simulink model "ConvertFrom_BFloat16_Ex2"  (R2023a)
settings: Solver=VariableStepAuto  StartTime=0.0  StopTime=1  RelTol=1e-3
undefined symbols (not defined in the file): AIE, i, L, ML, nsvh1369, xcvc2602
libraries: aieUtilities x2, vmcUtilities x1, dspsrcs4 x1
settings Model: Creator=sdegala  LastModifiedBy=robg

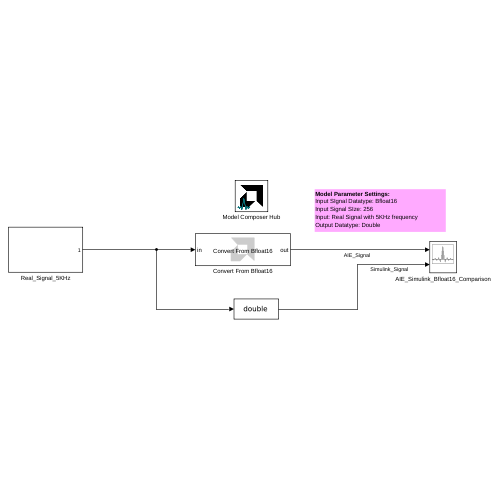
[thumbnail: Simulink's stored preview of the top-level diagram]
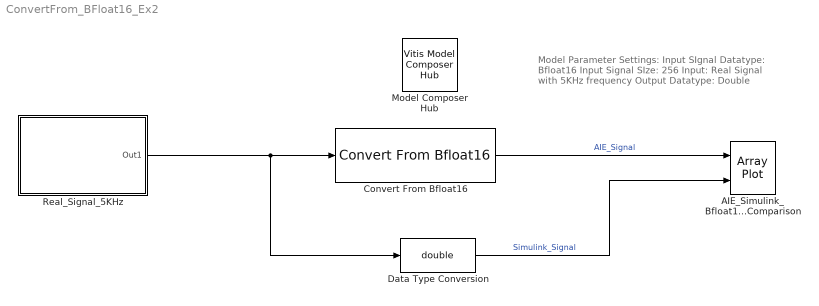
== system ConvertFrom_BFloat16_Ex2 ==
  note: Model Parameter Settings:
      | Input SIgnal Datatype: Bfloat16
      | Input Signal SIze: 256
      | Input: Real Signal with 5KHz frequency
      | Output Datatype: Double
  AIE_Simulink_Bfloat16_Comparison : ArrayPlot  NumInputPorts=2  WindowPosition=[1.000000,6.000000,1274.000000,655.000000,]  ScopeFrameLocation=window  PlotType=Line  YLimits=[-1.25,1.25]  ShowLegend=on  DefaultConfigurationName=dsp.scopes.ArrayPlotBlockSpecification
  Convert From Bfloat16 : aieUtilities/Convert From Bfloat16  OutputDataType=double
  Data Type Conversion : DataTypeConversion  OutDataTypeStr=double  SaturateOnIntegerOverflow=off  RndMeth=Floor
  Model Composer Hub : vmcUtilities/Vitis Model Composer Hub  Tag=genX  CodeGeneration=off  CompilationType=HDLCompilation  ExportTypeV2=IP Catalog  StartColumn=1  NumberOfColumns=1  TargetDirectory=./netlist  exportDesign=off  analyzeDesign=off  validateDesignOnHw=off  ExportType=AI Engines  IpVendor=xilinx.com  IpLibrary=hls  IpVersion=1.0  IpHWLanguage=Verilog  AieCompilerOptions={}  AieSimulatorOptions={}  CreateTestbench=on  TestbenchStackSize=10  RunRtlSim=off  RunCSim=off  RunAieSim=on  AieSimTimeout=50000  RunAieSimProfiling=off  LaunchVitisAnalyzer=off  PlotOutput=off  RunX86Sim=off  X86SimTimeout=10  GenHwImage=off  GenLibadfXo=off  GenHwValidationCode=off  PlatformType=Not Specified  HwSystemType=Baremetal  HwValidationTarget=hw  ProjDevice=xcvc2602-nsvh1369-1LHP-i-L  ProjDevicePart=xcvc2602-nsvh1369-1LHP-i-L  AIEType=AIE-ML  SamplePeriod=-1  ClockFrequency=200  DataPathParallelism=1  xilinxfamily=Kintex7  part=xc7k325t  speed=-3  package=fbg676  directory=./netlist  testbench=off  incr_netlist=off  synthesis_tool=Vivado  clock_wrapper=Clock Enables  dbl_ovrd=According to Block Masks  dcm_input_clock_period=10  sysclk_period=10  simulink_period=1  eval_field=0  LogFileName=/proj/xcoswmktg/robg/git/vmc_examples/gitent/Examples/AIENGINE/DSPlib/Dynamic_FFT/code/model_composer.log  NThreads=4
  Real_Signal_5KHz : Subsystem
  wires:
  Real_Signal_5KHz/1(Out1) -> Data Type Conversion/1, Convert From Bfloat16/1
  Convert From Bfloat16/1 -> AIE_Simulink_Bfloat16_Comparison/1  "AIE_Signal"
  Data Type Conversion/1 -> AIE_Simulink_Bfloat16_Comparison/2  "Simulink_Signal"

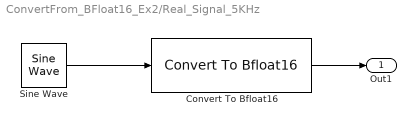
== system ConvertFrom_BFloat16_Ex2/Real_Signal_5KHz ==
  Convert To Bfloat16 : aieUtilities/Convert To Bfloat16
  Sine Wave : dspsrcs4/Sine Wave  Amplitude=1  Frequency=5e3  Phase=0  SampleMode=Discrete  OutComplex=Real  CompMethod=Trigonometric fcn  TableSize=Speed  SampleTime=1/20e3  SamplesPerFrame=256  ResetState=Restart at time zero  OutputFrames=off  dataType=single  wordLen=16  udDataType=sfix(16)  fracBitsMode=User-defined  numFracBits=0  OutDataTypeStr=single  LastOutDataTypeStr=single
  Out1 : Outport
  wires:
  Sine Wave/1 -> Convert To Bfloat16/1
  Convert To Bfloat16/1 -> Out1/1
